simulink model "ClosedLoopTest"  (R2023a)
settings: Solver=VariableStepAuto  StartTime=0.0  StopTime=500  RelTol=1e-3
undefined symbols (not defined in the file): B, I, J, Ke, Kt, La, Ra, RW_omega_max, T_ext, T_max
libraries: simulink_extras x7, matrix_library x5, slpidlib x3, simulink x2, vrlib x2, aerolibutil x1
settings Model: Creator=Personal  LastModifiedBy=Personal
settings OptimizationCC: ReuseModelBlockBuffer=off
settings DebuggingCC: UnderSpecifiedDimensionMsg=warning

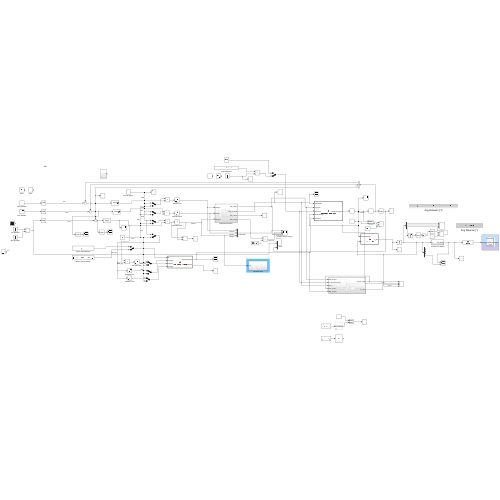
[thumbnail: Simulink's stored preview of the top-level diagram]
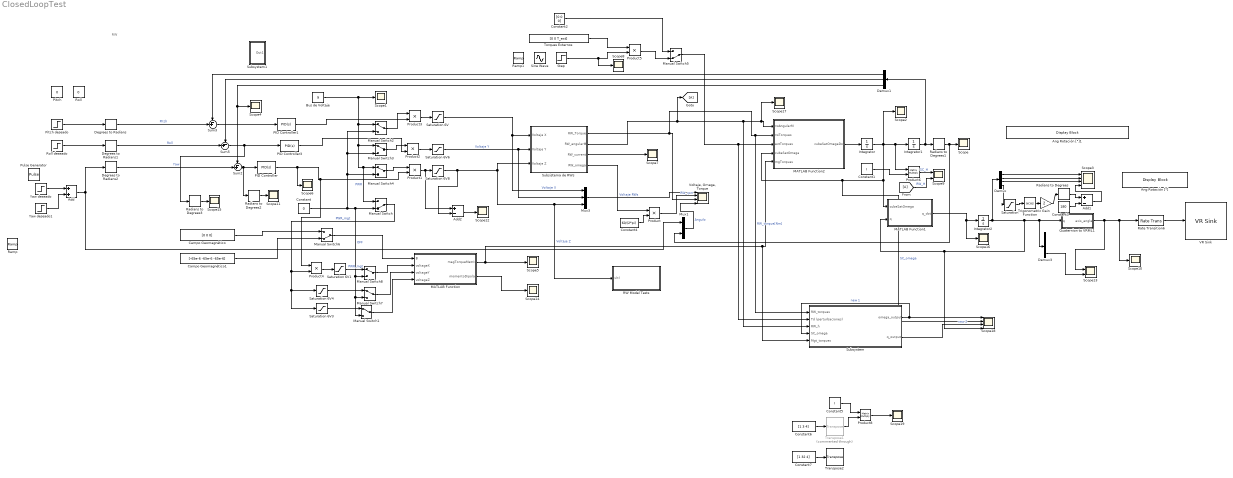
== system ClosedLoopTest ==
  note: RW
  Add : Sum
  Add1 : Sum  Inputs=+-
  Add2 : Sum  Inputs=+-
  Ang Rotación [°] : DisplayBlock  LabelPosition=Hide  Transparency=1
  Ang Rotación [°]1 : DisplayBlock  LabelPosition=Hide  Transparency=1
  Bus de Voltaje : Constant  Value=9
  Campo Geomagnético : Constant  Value=[0 0 0]
  Campo Geomagnético1 : Constant  Value=[-65e-6 -65e-6 -65e-6]
  Constant : Constant  Value=0
  Constant1 : Constant  Value=I
  Constant2 : Constant  Value=[0 0 0]
  Constant3 : Constant  Value=180
  Constant4 : Constant  Value=60/(2*pi)
  Constant5 : Constant  Value=I
  Constant6 : Constant  Value=[1 3 4]
  Constant7 : Constant  Value=[1 32 4]
  Degrees to Radians : simulink_extras/Transformations/Degrees to Radians
  Degrees to Radians1 : simulink_extras/Transformations/Degrees to Radians
  Degrees to Radians2 : simulink_extras/Transformations/Degrees to Radians
  Demux : Demux
  Demux1 : Demux  Outputs=3
  Demux3 : Demux
  From : From
  Gain : Gain  Gain=2
  Goto : Goto
  Integrator : Integrator  InitialCondition=[0 0 0]
  Integrator1 : Integrator  InitialCondition=[0 0 0]
  Integrator2 : Integrator  InitialCondition=[0 0 0 1]
  MATLAB Function : MATLAB Function  TreatAsAtomicUnit=on
  MATLAB Function1 : MATLAB Function  TreatAsAtomicUnit=on
  MATLAB Function2 : MATLAB Function  TreatAsAtomicUnit=on
  Manual Switch : ManualSwitch  CurrentSetting=0
  Manual Switch{1..4,7..8} (6 alike) : ManualSwitch
  Manual Switch5 : ManualSwitch  CurrentSetting=0
  Manual Switch6 : ManualSwitch  CurrentSetting=0
  Mux1 : Mux  Inputs=2
  Mux3 : Mux  Inputs=3
  PID Controller : slpidlib/PID Controller  Controller=PID  Form=Parallel  TimeDomain=Continuous-time  UseExternalTs=off  SampleTime=-1  IntegratorMethod=Forward Euler  FilterMethod=Forward Euler  ControllerParametersSource=internal  P=4500  I=800  UseKiTs=off  D=8000  N=100  UseFilter=on  TunerSelectOption=Transfer Function Based (PID Tuner App)  InitialConditionSource=internal  InitialConditionForIntegrator=0  InitialConditionForFilter=0  DifferentiatorICPrevScaledInput=0  ExternalReset=none  TrackingMode=off  Kt=1  LimitOutput=off  SatLimitsSource=internal  UpperSaturationLimit=1  LowerSaturationLimit=-1  LinearizeAsGain=on  AntiWindupMode=none  Kb=1  LimitIntegrator=off  UpperIntegratorSaturationLimit=inf  LowerIntegratorSaturationLimit=-inf  POutMin=[]  POutMax=[]  IOutMin=[]  IOutMax=[]  DOutMin=[]  DOutMax=[]  NOutMin=[]  NOutMax=[]  SumOutMin=[]  SumOutMax=[]  SaturationOutMin=[]  SaturationOutMax=[]  PParamMin=[]  PParamMax=[]  IParamMin=[]  IParamMax=[]  DParamMin=[]  DParamMax=[]  NParamMin=[]  NParamMax=[]  KbParamMin=[]  KbParamMax=[]  KtParamMin=[]  KtParamMax=[]  KbOutMin=[]  KbOutMax=[]  KtOutMin=[]  KtOutMax=[]  IntegratorOutMin=[]  IntegratorOutMax=[]  FilterOutMin=[]  FilterOutMax=[]  SumI1OutMin=[]  SumI1OutMax=[]  SumI2OutMin=[]  SumI2OutMax=[]  SumI3OutMin=[]  SumI3OutMax=[]  SumI4OutMin=[]  SumI4OutMax=[]  SumDOutMin=[]  SumDOutMax=[]  DifferentiatorOutMin=[]  DifferentiatorOutMax=[]  FilterDiffOutCoefMin=[]  FilterDiffOutCoefMax=[]  ReciprocalOutMin=[]  ReciprocalOutMax=[]  SumDenOutMin=[]  SumDenOutMax=[]  SumNumOutMin=[]  SumNumOutMax=[]  DivideOutMin=[]  DivideOutMax=[]  UdiffTsProdOutMin=[]  UdiffTsProdOutMax=[]  NTsProdOutMin=[]  NTsProdOutMax=[]  UintegralTsProdOutMin=[]  UintegralTsProdOutMax=[]  UngainTsProdOutMin=[]  UngainTsProdOutMax=[]  ClampingZeroOutDataTypeStr=Inherit: Inherit via back propagation  ClampingZeroOutMin=[]  ClampingZeroOutMax=[]  FilterDenConstantOutDataTypeStr=Inherit: Inherit via back propagation  FilterDenConstantOutMin=[]  FilterDenConstantOutMax=[]  PCopyOutDataTypeStr=Inherit: Inherit via back propagation  PCopyOutMin=[]  PCopyOutMax=[]  NCopyOutDataTypeStr=Inherit: Inherit via back propagation  NCopyOutMin=[]  NCopyOutMax=[]  IntegratorContinuousStateAttributes=''  IntegratorStateMustResolveToSignalObject=off  IntegratorRTWStateStorageClass=Auto  FilterContinuousStateAttributes=''  FilterStateMustResolveToSignalObject=off  FilterRTWStateStorageClass=Auto  ParallelPVariant=InternalParameters  IdealPVariant=Disabled  IVariant=InternalParameters  DVariant=InternalParameters  IntegratorVariant=Continuous  SatVariant=Disabled  AWVariant=Passthrough  PCopyVariant=Disabled  TRVariant=Disabled  FdbkBlocksVariant=Forward  IdealPFdbkVariant=Disabled  SatFdbkVariant=Disabled  DerivativeFilterVariant=ContFilter  NVariant=InternalParameters  NCopyVariant=Disabled  FilterICVariant=InternalICsFilter  IntegratorICVariant=InternalICs  ExternalResetVariant=Disabled  TRSumVariant=Passthrough  SumFdbkVariant=Disabled  SumVariant=Sum_PID  TsampFilterVariant=InternalTs  TsampNgainVariant=Passthrough  TsampIntegralVariant=Disabled_SignalSpec  ExternalSaturationOutDataTypeStr=Inherit: Same as second input
  PID Controller1 : slpidlib/PID Controller  Controller=PID  Form=Parallel  TimeDomain=Continuous-time  UseExternalTs=off  SampleTime=-1  IntegratorMethod=Forward Euler  FilterMethod=Forward Euler  ControllerParametersSource=internal  P=4500  I=800  UseKiTs=off  D=8000  N=100  UseFilter=on  TunerSelectOption=Transfer Function Based (PID Tuner App)  InitialConditionSource=internal  InitialConditionForIntegrator=0  InitialConditionForFilter=0  DifferentiatorICPrevScaledInput=0  ExternalReset=none  TrackingMode=off  Kt=1  LimitOutput=on  SatLimitsSource=internal  UpperSaturationLimit=1  LowerSaturationLimit=-1  LinearizeAsGain=on  AntiWindupMode=none  Kb=1  LimitIntegrator=off  UpperIntegratorSaturationLimit=inf  LowerIntegratorSaturationLimit=-inf  POutMin=[]  POutMax=[]  IOutMin=[]  IOutMax=[]  DOutMin=[]  DOutMax=[]  NOutMin=[]  NOutMax=[]  SumOutMin=[]  SumOutMax=[]  SaturationOutMin=[]  SaturationOutMax=[]  PParamMin=[]  PParamMax=[]  IParamMin=[]  IParamMax=[]  DParamMin=[]  DParamMax=[]  NParamMin=[]  NParamMax=[]  KbParamMin=[]  KbParamMax=[]  KtParamMin=[]  KtParamMax=[]  KbOutMin=[]  KbOutMax=[]  KtOutMin=[]  KtOutMax=[]  IntegratorOutMin=[]  IntegratorOutMax=[]  FilterOutMin=[]  FilterOutMax=[]  SumI1OutMin=[]  SumI1OutMax=[]  SumI2OutMin=[]  SumI2OutMax=[]  SumI3OutMin=[]  SumI3OutMax=[]  SumI4OutMin=[]  SumI4OutMax=[]  SumDOutMin=[]  SumDOutMax=[]  DifferentiatorOutMin=[]  DifferentiatorOutMax=[]  FilterDiffOutCoefMin=[]  FilterDiffOutCoefMax=[]  ReciprocalOutMin=[]  ReciprocalOutMax=[]  SumDenOutMin=[]  SumDenOutMax=[]  SumNumOutMin=[]  SumNumOutMax=[]  DivideOutMin=[]  DivideOutMax=[]  UdiffTsProdOutMin=[]  UdiffTsProdOutMax=[]  NTsProdOutMin=[]  NTsProdOutMax=[]  UintegralTsProdOutMin=[]  UintegralTsProdOutMax=[]  UngainTsProdOutMin=[]  UngainTsProdOutMax=[]  ClampingZeroOutDataTypeStr=Inherit: Inherit via back propagation  ClampingZeroOutMin=[]  ClampingZeroOutMax=[]  FilterDenConstantOutDataTypeStr=Inherit: Inherit via back propagation  FilterDenConstantOutMin=[]  FilterDenConstantOutMax=[]  PCopyOutDataTypeStr=Inherit: Inherit via back propagation  PCopyOutMin=[]  PCopyOutMax=[]  NCopyOutDataTypeStr=Inherit: Inherit via back propagation  NCopyOutMin=[]  NCopyOutMax=[]  IntegratorContinuousStateAttributes=''  IntegratorStateMustResolveToSignalObject=off  IntegratorRTWStateStorageClass=Auto  FilterContinuousStateAttributes=''  FilterStateMustResolveToSignalObject=off  FilterRTWStateStorageClass=Auto  ParallelPVariant=InternalParameters  IdealPVariant=Disabled  IVariant=InternalParameters  DVariant=InternalParameters  IntegratorVariant=Continuous  SatVariant=Enabled  AWVariant=Passthrough  PCopyVariant=Disabled  TRVariant=Disabled  FdbkBlocksVariant=Forward  IdealPFdbkVariant=Disabled  SatFdbkVariant=Disabled  DerivativeFilterVariant=ContFilter  NVariant=InternalParameters  NCopyVariant=Disabled  FilterICVariant=InternalICsFilter  IntegratorICVariant=InternalICs  ExternalResetVariant=Disabled  TRSumVariant=Passthrough  SumFdbkVariant=Disabled  SumVariant=Sum_PID  TsampFilterVariant=InternalTs  TsampNgainVariant=Passthrough  TsampIntegralVariant=Disabled_SignalSpec  ExternalSaturationOutDataTypeStr=Inherit: Same as second input
  PID Controller3 : slpidlib/PID Controller  Controller=PID  Form=Parallel  TimeDomain=Continuous-time  UseExternalTs=off  SampleTime=-1  IntegratorMethod=Forward Euler  FilterMethod=Forward Euler  ControllerParametersSource=internal  P=4500  I=800  UseKiTs=off  D=8000  N=100  UseFilter=on  TunerSelectOption=Transfer Function Based (PID Tuner App)  InitialConditionSource=internal  InitialConditionForIntegrator=0  InitialConditionForFilter=0  DifferentiatorICPrevScaledInput=0  ExternalReset=none  TrackingMode=off  Kt=1  LimitOutput=on  SatLimitsSource=internal  UpperSaturationLimit=1  LowerSaturationLimit=-1  LinearizeAsGain=on  AntiWindupMode=none  Kb=1  LimitIntegrator=off  UpperIntegratorSaturationLimit=inf  LowerIntegratorSaturationLimit=-inf  POutMin=[]  POutMax=[]  IOutMin=[]  IOutMax=[]  DOutMin=[]  DOutMax=[]  NOutMin=[]  NOutMax=[]  SumOutMin=[]  SumOutMax=[]  SaturationOutMin=[]  SaturationOutMax=[]  PParamMin=[]  PParamMax=[]  IParamMin=[]  IParamMax=[]  DParamMin=[]  DParamMax=[]  NParamMin=[]  NParamMax=[]  KbParamMin=[]  KbParamMax=[]  KtParamMin=[]  KtParamMax=[]  KbOutMin=[]  KbOutMax=[]  KtOutMin=[]  KtOutMax=[]  IntegratorOutMin=[]  IntegratorOutMax=[]  FilterOutMin=[]  FilterOutMax=[]  SumI1OutMin=[]  SumI1OutMax=[]  SumI2OutMin=[]  SumI2OutMax=[]  SumI3OutMin=[]  SumI3OutMax=[]  SumI4OutMin=[]  SumI4OutMax=[]  SumDOutMin=[]  SumDOutMax=[]  DifferentiatorOutMin=[]  DifferentiatorOutMax=[]  FilterDiffOutCoefMin=[]  FilterDiffOutCoefMax=[]  ReciprocalOutMin=[]  ReciprocalOutMax=[]  SumDenOutMin=[]  SumDenOutMax=[]  SumNumOutMin=[]  SumNumOutMax=[]  DivideOutMin=[]  DivideOutMax=[]  UdiffTsProdOutMin=[]  UdiffTsProdOutMax=[]  NTsProdOutMin=[]  NTsProdOutMax=[]  UintegralTsProdOutMin=[]  UintegralTsProdOutMax=[]  UngainTsProdOutMin=[]  UngainTsProdOutMax=[]  ClampingZeroOutDataTypeStr=Inherit: Inherit via back propagation  ClampingZeroOutMin=[]  ClampingZeroOutMax=[]  FilterDenConstantOutDataTypeStr=Inherit: Inherit via back propagation  FilterDenConstantOutMin=[]  FilterDenConstantOutMax=[]  PCopyOutDataTypeStr=Inherit: Inherit via back propagation  PCopyOutMin=[]  PCopyOutMax=[]  NCopyOutDataTypeStr=Inherit: Inherit via back propagation  NCopyOutMin=[]  NCopyOutMax=[]  IntegratorContinuousStateAttributes=''  IntegratorStateMustResolveToSignalObject=off  IntegratorRTWStateStorageClass=Auto  FilterContinuousStateAttributes=''  FilterStateMustResolveToSignalObject=off  FilterRTWStateStorageClass=Auto  ParallelPVariant=InternalParameters  IdealPVariant=Disabled  IVariant=InternalParameters  DVariant=InternalParameters  IntegratorVariant=Continuous  SatVariant=Enabled  AWVariant=Passthrough  PCopyVariant=Disabled  TRVariant=Disabled  FdbkBlocksVariant=Forward  IdealPFdbkVariant=Disabled  SatFdbkVariant=Disabled  DerivativeFilterVariant=ContFilter  NVariant=InternalParameters  NCopyVariant=Disabled  FilterICVariant=InternalICsFilter  IntegratorICVariant=InternalICs  ExternalResetVariant=Disabled  TRSumVariant=Passthrough  SumFdbkVariant=Disabled  SumVariant=Sum_PID  TsampFilterVariant=InternalTs  TsampNgainVariant=Passthrough  TsampIntegralVariant=Disabled_SignalSpec  ExternalSaturationOutDataTypeStr=Inherit: Same as second input
  Pitch : Constant  Value=0
  Pitch deseado : Step  Time=5  After=0  SampleTime=0
  Product{,1..5} (6 alike) : Product
  Product6 : Product  Multiplication=Matrix(*)
  Product8 : Product  Multiplication=Matrix(*)
  Pulse Generator : DiscretePulseGenerator  PulseType=Time based  Amplitude=45  Period=20  PulseWidth=50
  Quaternion to VRML1 : Subsystem
  RW Model Tests : Subsystem
  Radians to Degrees{,1..3} (4 alike) : simulink_extras/Transformations/Radians to Degrees
  Ramp : simulink/Sources/Ramp  slope=5  start=0  InitialOutput=0
  Ramp1 : simulink/Sources/Ramp  slope=2  start=3  InitialOutput=0
  Rate Transition6 : RateTransition
  Roll : Constant  Value=0
  Roll deseado : Step  Time=5  After=0  SampleTime=0
  Saturation : Saturate  UpperLimit=1  LowerLimit=-1
  Saturation 6V{,3,6,8} (4 alike) : Saturate  UpperLimit=6  LowerLimit=-6
  Saturation 6V1 : Saturate  UpperLimit=5  LowerLimit=-5
  Saturation 6V4 : Saturate  UpperLimit=2  LowerLimit=-6
  Scope{,1..2,4..8,10..12,14..17,19} (16 alike) : Scope
  Scope13 : Scope  NumInputPorts=2
  Scope18 : Scope  NumInputPorts=4
  Scope3 : Scope  NumInputPorts=4
  Scope9 : Scope  NumInputPorts=2
  Sine Wave : Sin  Amplitude=1.5  Frequency=0.01  SampleTime=0
  Step : Step  Time=0  After=100  SampleTime=0
  "Subsistema de RWs  " : Subsystem
  Subsystem : Subsystem
  Subsystem1 : Subsystem
  Sum2 : Sum  Inputs=-+|
  Sum3 : Sum  Inputs=-+|
  Sum5 : Sum  Inputs=-+|
  Torques Externos : Constant  Value=[0 0 T_ext]
  Transpose1 : matrix_library/Transpose  Commented=through
  Transpose2 : matrix_library/Transpose
  Trigonometric Function : Trigonometry  Operator=acos
  VR Sink : vrlib/VR Sink  InstantiateOnLoad=on  SampleTime=0.1  ViewEnable=on  RemoteChange=off  RemoteView=off  FieldsWritten=STLB_Transform.rotation.4.1.1.double  WorldFileName=EscenarioCubeSat.x3d  AutoView=off  VideoDimensions=[]  AllowVariableSize=off
  "Voltaje, Omega, Torque" : Scope  NumInputPorts=4
  Yaw deseado : Step  Time=5  After=45  SampleTime=0
  Yaw deseado1 : Step  Time=15  After=0  SampleTime=0
  wires:
  Saturation 6V/1 -> Mux3/1, "Subsistema de RWs  "/1(Voltaje X)  "Voltaje X"
  Saturation 6V6/1 -> "Subsistema de RWs  "/2(Voltaje Y), Mux3/2  "Voltaje Y"
  Saturation 6V8/1 -> Add2/2, "Subsistema de RWs  "/3(Voltaje Z), RW Model Tests/1(v(t)), Mux3/3  "Voltaje Z"
  MATLAB Function2/1(cubeSatOmegaDot) -> Integrator/1
  Integrator/1 -> Product6/1, Integrator1/1, Scope18/2, MATLAB Function2/4(cubeSatOmega), MATLAB Function1/1(cubeSatOmega), Scope2/1  "SC_omega"
  Integrator1/1 -> Demux1/1, Radians to Degrees1/1
  MATLAB Function/1(magTorqueMatrix) -> Subsystem/5(Mgt_torques), MATLAB Function2/5(mgTorques), Scope5/1
  Constant/1 -> Manual Switch2/2, Manual Switch3/2, Manual Switch4/2, Manual Switch1/2, Manual Switch7/2, Manual Switch8/2, Manual Switch/2  "OFF"
  Saturation 6V3/1 -> Manual Switch1/1
  Manual Switch1/1 -> MATLAB Function/4(voltageZ)
  Manual Switch5/1 -> Subsystem/2(Td (perturbaciones)), MATLAB Function2/3(extTorques)
  Constant2/1 -> Manual Switch5/1
  Manual Switch6/1 -> MATLAB Function/1(B)
  Campo Geomagnético/1 -> Manual Switch6/1
  Campo Geomagnético1/1 -> Manual Switch6/2
  Saturation 6V4/1 -> Manual Switch7/1
  Manual Switch/1 -> Saturation 6V4/1, Saturation 6V3/1, Product4/2  "PWR_mgt"
  Manual Switch8/1 -> MATLAB Function/2(voltageX)
  Manual Switch7/1 -> MATLAB Function/3(voltageY)
  MATLAB Function1/1(q_dot) -> Scope16/1, Integrator2/1
  Integrator2/1 -> Quaternion to VRML1/1(q), Demux3/1, Scope18/4, MATLAB Function1/2(q), Demux/1
  Demux/1 -> Scope3/1
  Demux/2 -> Scope3/2
  Demux/3 -> Scope3/3
  Radians to Degrees/1 -> Add1/1
  Radians to Degrees1/1 -> Mux1/2, Scope/1
  Demux/4 -> Saturation/1
  Trigonometric Function/1 -> Gain/1
  Gain/1 -> Radians to Degrees/1
  Quaternion to VRML1/1(axis_angle) -> Scope13/1, Scope10/1, Rate Transition6/1
  Constant3/1 -> Add1/2
  Add1/1 -> Scope3/4
  Bus de Voltaje/1 -> Manual Switch2/1, Manual Switch3/1, Manual Switch/1, Manual Switch4/1, Scope1/1  "PWR"
  MATLAB Function/2(momentoDipolar) -> Scope14/1
  Constant4/1 -> Product/2
  Product/1 -> "Voltaje, Omega, Torque"/2  "RW_rpm"
  Demux3/4 -> Scope13/2
  Rate Transition6/1 -> VR Sink/1
  Saturation/1 -> Trigonometric Function/1
  Add/1 -> Degrees to Radians2/1, Mux1/1
  Degrees to Radians/1 -> Sum3/2  "Pitch"
  Degrees to Radians2/1 -> Sum2/2  "Yaw"
  Degrees to Radians1/1 -> Sum5/2  "Roll"
  Demux1/1 -> Sum3/1
  Demux1/2 -> Sum5/1
  Demux1/3 -> Scope4/1, Sum2/1
  Manual Switch4/1 -> Product1/1
  Product1/1 -> Add2/1, Saturation 6V8/1
  Sum3/1 -> PID Controller1/1
  Product3/1 -> Saturation 6V/1
  Product2/1 -> Saturation 6V6/1
  Manual Switch3/1 -> Product2/1
  Manual Switch2/1 -> Product3/1
  PID Controller1/1 -> Product3/2
  PID Controller3/1 -> Product2/2
  Radians to Degrees2/1 -> Scope11/1
  Product4/1 -> Saturation 6V1/1
  Saturation 6V1/1 -> Manual Switch8/1  "PWR_mgt"
  PID Controller/1 -> Scope6/1, Product1/2, Product4/1
  Sum2/1 -> PID Controller/1, Radians to Degrees2/1
  Torques Externos/1 -> Product5/1
  Step/1 -> Scope8/1, Product5/2
  Product5/1 -> Manual Switch5/2
  Sum5/1 -> Radians to Degrees3/1, PID Controller3/1
  Radians to Degrees3/1 -> Scope15/1
  Roll deseado/1 -> Degrees to Radians1/1
  Pitch deseado/1 -> Degrees to Radians/1
  Mux3/1 -> "Voltaje, Omega, Torque"/1  "Voltaje RWs"
  "Subsistema de RWs  "/2(RW_angularM) -> Goto/1, Subsystem/3(RW_h), Scope17/1, MATLAB Function2/1(rwAngularM)
  "Subsistema de RWs  "/4(RW_omega) -> Product/1
  "Subsistema de RWs  "/1(RW_Torque) -> Subsystem/1(RW_torques), MATLAB Function2/2(rwTorques), "Voltaje, Omega, Torque"/3  "RW_torque[Nm]"
  "Subsistema de RWs  "/3(RW_current) -> Scope7/1
  Mux1/1 -> "Voltaje, Omega, Torque"/4  "Angulo"
  Constant1/1 -> Product6/2
  Product6/1 -> Scope9/1  "SC_H"
  From/1 -> Scope9/2  "RW_H"
  Yaw deseado/1 -> Add/1
  Yaw deseado1/1 -> Add/2
  Add2/1 -> Scope12/1
  Subsystem/1(omega_output) -> Scope18/1, Subsystem/4(SC_omega)  "new 1"
  Subsystem/2(q_output) -> Scope18/3  "new 2"
  Constant5/1 -> Product8/1
  Transpose1/1 -> Product8/2
  Constant6/1 -> Transpose1/1
  Product8/1 -> Scope19/1
  Constant7/1 -> Transpose2/1

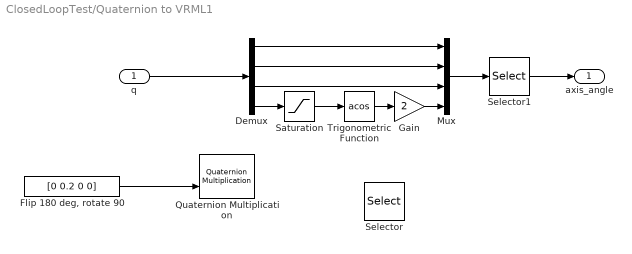
== system ClosedLoopTest/Quaternion to VRML1 ==
  q : Inport
  Demux : Demux
  "Flip 180 deg, rotate 90" : Constant  Value=[0 0.2 0 0]
  Gain : Gain  Gain=2
  Mux : Mux
  Quaternion Multiplication : aerolibutil/Quaternion Multiplication
  Saturation : Saturate  UpperLimit=1  LowerLimit=-1  ZeroCross=off
  Selector : Selector  InputPortWidth=3  IndexOptions=Index vector (dialog)  Indices=[1 3]  OutputSizes=1
  Selector1 : Selector  InputPortWidth=4  IndexOptions=Index vector (dialog)  Indices=[2 3 1 4]  OutputSizes=1
  Trigonometric Function : Trigonometry  Operator=acos
  axis_angle : Outport  VectorParamsAs1DForOutWhenUnconnected=off
  wires:
  Demux/2 -> Mux/2
  "Flip 180 deg, rotate 90"/1 -> Quaternion Multiplication/2
  q/1 -> Demux/1
  Demux/1 -> Mux/1
  Mux/1 -> Selector1/1
  Selector1/1 -> axis_angle/1
  Trigonometric Function/1 -> Gain/1
  Gain/1 -> Mux/4
  Demux/3 -> Mux/3
  Saturation/1 -> Trigonometric Function/1
  Demux/4 -> Saturation/1

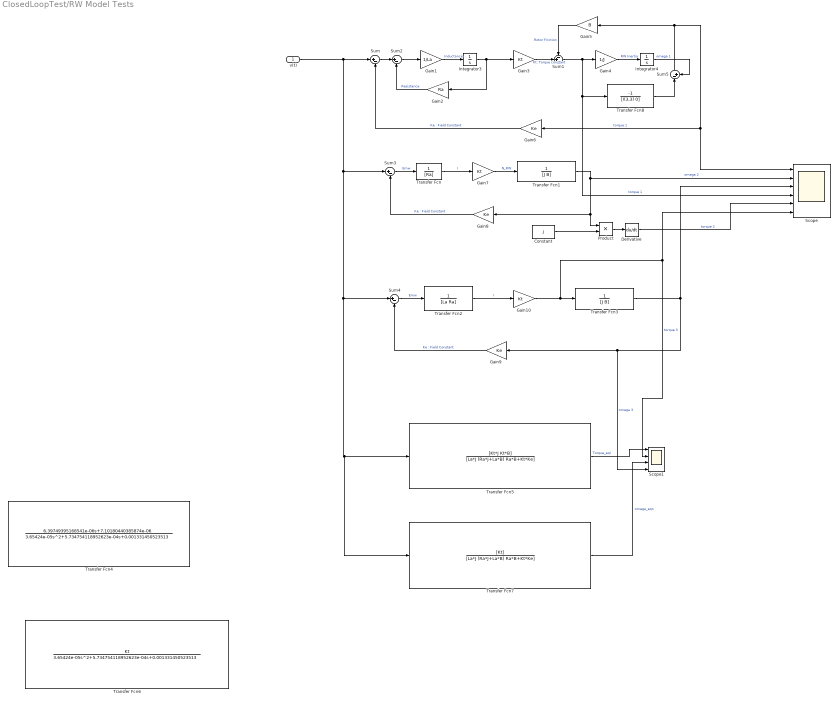
== system ClosedLoopTest/RW Model Tests ==
  v(t) : Inport
  Constant : Constant  Value=J
  Derivative : Derivative
  Gain1 : Gain  Gain=1/La
  Gain10 : Gain  Gain=Kt
  Gain2 : Gain  Gain=Ra
  Gain3 : Gain  Gain=Kt
  Gain4 : Gain  Gain=1/J
  Gain5 : Gain  Gain=B
  Gain6 : Gain  Gain=Ke
  Gain7 : Gain  Gain=Kt
  Gain8 : Gain  Gain=Ke
  Gain9 : Gain  Gain=Ke
  Integrator3 : Integrator
  Integrator4 : Integrator
  Product : Product
  Scope : Scope  NumInputPorts=6
  Scope1 : Scope  NumInputPorts=4
  Sum{,2..4} (4 alike) : Sum  Inputs=|+-
  Sum1 : Sum  Inputs=-+|
  Sum5 : Sum  Inputs=|-+
  Transfer Fcn : TransferFcn  Denominator=[Ra]
  Transfer Fcn1 : TransferFcn  Denominator=[J B]
  Transfer Fcn2 : TransferFcn  Denominator=[La Ra]
  Transfer Fcn3 : TransferFcn  Denominator=[J B]
  Transfer Fcn4 : TransferFcn  Numerator=[6.39749395168541e-06 7.10180440385874e-06]  Denominator=[3.65424e-05 5.734754118952623e-04 0.001331450523513]
  Transfer Fcn5 : TransferFcn  Numerator=[Kt*J Kt*B]  Denominator=[La*J (Ra*J+La*B) Ra*B+Kt*Ke]
  Transfer Fcn6 : TransferFcn  Numerator=Kt  Denominator=[3.65424e-05 5.734754118952623e-04 0.001331450523513]
  Transfer Fcn7 : TransferFcn  Numerator=[Kt]  Denominator=[La*J (Ra*J+La*B) Ra*B+Kt*Ke]
  Transfer Fcn8 : TransferFcn  Numerator=[-1]  Denominator=[I(3,3) 0]
  wires:
  Sum1/1 -> Gain4/1, Transfer Fcn8/1, Scope/4  "torque 1"
  Derivative/1 -> Scope/5  "torque 2"
  Transfer Fcn3/1 -> Scope/3, Gain9/1, Scope1/4  "omega 3"
  Gain10/1 -> Transfer Fcn3/1, Scope/6, Scope1/2  "torque 3"
  Transfer Fcn2/1 -> Gain10/1  "I"
  Gain9/1 -> Sum4/2  "Ke : Field Constant"
  Sum4/1 -> Transfer Fcn2/1  "Emw"
  Gain2/1 -> Sum2/2  "Resistance"
  Integrator3/1 -> Gain2/1, Gain3/1
  Gain6/1 -> Sum/2  "Ke : Field Constant"
  Gain5/1 -> Sum1/1  "Rotor Friction"
  Sum2/1 -> Gain1/1
  Integrator4/1 -> Sum5/2  "omega 1"
  Gain4/1 -> Integrator4/1  "RW Inertia"
  Gain1/1 -> Integrator3/1  "Inductance"
  Gain3/1 -> Sum1/2  "Kt: Torque constant"
  Sum/1 -> Sum2/1
  v(t)/1 -> Transfer Fcn7/1, Transfer Fcn5/1, Sum4/1, Sum3/1, Sum/1
  Sum3/1 -> Transfer Fcn/1  "Emw"
  Gain7/1 -> Transfer Fcn1/1  "N_RW"
  Transfer Fcn/1 -> Gain7/1  "I"
  Transfer Fcn1/1 -> Product/1, Gain8/1, Scope/2  "omega 2"
  Gain8/1 -> Sum3/2  "Ke : Field Constant"
  Product/1 -> Derivative/1
  Constant/1 -> Product/2
  Transfer Fcn5/1 -> Scope1/1  "Torque_eqI"
  Transfer Fcn7/1 -> Scope1/3  "omega_eqn"
  Transfer Fcn8/1 -> Sum5/1
  Sum5/1 -> Gain5/1, Scope/1, Gain6/1  "torque 1"

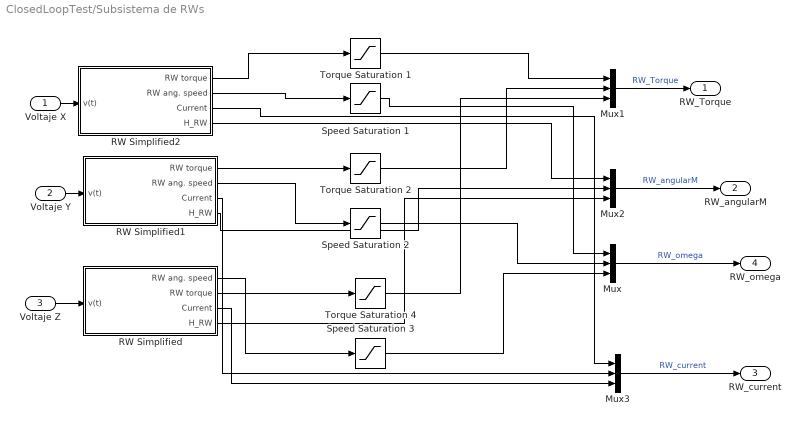
== system ClosedLoopTest/Subsistema de RWs   ==
  Voltaje X : Inport
  Voltaje Y : Inport  Port=2
  Voltaje Z : Inport  Port=3
  Mux{,1..3} (4 alike) : Mux  Inputs=3
  RW Simplified : Subsystem
  RW Simplified1 : Subsystem
  RW Simplified2 : Subsystem
  Speed Saturation 1 : Saturate  UpperLimit=RW_omega_max  LowerLimit=-RW_omega_max
  Speed Saturation 2 : Saturate  UpperLimit=RW_omega_max  LowerLimit=-RW_omega_max
  Speed Saturation 3 : Saturate  UpperLimit=RW_omega_max  LowerLimit=-RW_omega_max
  Torque Saturation 1 : Saturate  UpperLimit=T_max  LowerLimit=-T_max
  Torque Saturation 2 : Saturate  UpperLimit=T_max  LowerLimit=-T_max
  Torque Saturation 4 : Saturate  UpperLimit=T_max  LowerLimit=-T_max
  RW_Torque : Outport
  RW_angularM : Outport  Port=2
  RW_current : Outport  Port=3
  RW_omega : Outport  Port=4
  wires:
  RW Simplified/2(RW torque) -> Torque Saturation 4/1
  RW Simplified2/1(RW torque) -> Torque Saturation 1/1
  Torque Saturation 4/1 -> Mux1/3
  Voltaje Z/1 -> RW Simplified/1(v(t))
  Speed Saturation 2/1 -> Mux/2
  RW Simplified1/1(RW torque) -> Torque Saturation 2/1
  RW Simplified/4(H_RW) -> Mux2/3
  Mux1/1 -> RW_Torque/1  "RW_Torque"
  Voltaje X/1 -> RW Simplified2/1(v(t))
  Speed Saturation 1/1 -> Mux/1
  RW Simplified1/4(H_RW) -> Mux2/2
  Speed Saturation 3/1 -> Mux/3
  Voltaje Y/1 -> RW Simplified1/1(v(t))
  RW Simplified1/2(RW ang. speed) -> Speed Saturation 2/1
  RW Simplified2/4(H_RW) -> Mux2/1
  RW Simplified2/2(RW ang. speed) -> Speed Saturation 1/1
  RW Simplified/1(RW ang. speed) -> Speed Saturation 3/1
  Torque Saturation 2/1 -> Mux1/2
  Mux2/1 -> RW_angularM/1  "RW_angularM"
  Torque Saturation 1/1 -> Mux1/1
  Mux/1 -> RW_omega/1  "RW_omega"
  RW Simplified/3(Current) -> Mux3/3
  RW Simplified1/3(Current) -> Mux3/2
  Mux3/1 -> RW_current/1  "RW_current"
  RW Simplified2/3(Current) -> Mux3/1

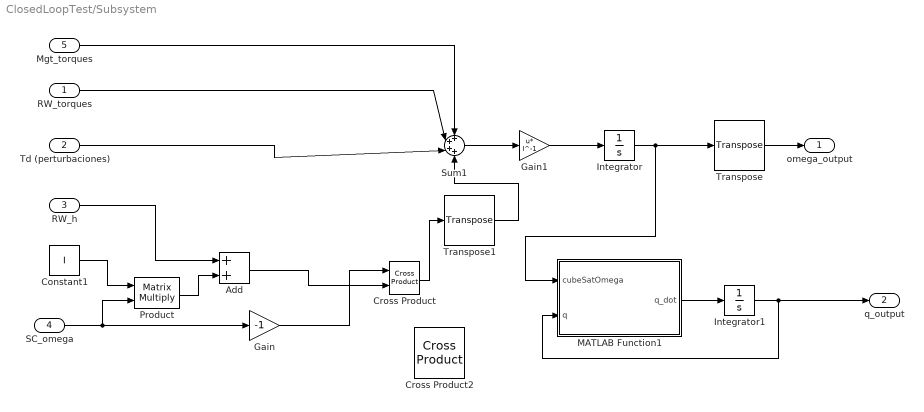
== system ClosedLoopTest/Subsystem ==
  RW_torques : Inport
  Td (perturbaciones) : Inport  Port=2
  RW_h : Inport  Port=3
  SC_omega : Inport  Port=4
  Mgt_torques : Inport  Port=5
  Add : Sum
  Constant1 : Constant  Value=I
  Cross Product : vrlib/Utilities/Cross Product
  Cross Product2 : matrix_library/Cross Product
  Gain : Gain  Gain=-1
  Gain1 : Gain  Gain=I^-1  Multiplication=Matrix(u*K)
  Integrator : Integrator  InitialCondition=[0 0 0]
  Integrator1 : Integrator  InitialCondition=[0 0 0 1]
  MATLAB Function1 : MATLAB Function  TreatAsAtomicUnit=on
  Product : Product  Multiplication=Matrix(*)
  Sum1 : Sum  Inputs=++++
  Transpose : matrix_library/Transpose
  Transpose1 : matrix_library/Transpose
  omega_output : Outport
  q_output : Outport  Port=2
  wires:
  RW_torques/1 -> Sum1/2
  Td (perturbaciones)/1 -> Sum1/3
  Integrator1/1 -> MATLAB Function1/2(q), q_output/1
  Constant1/1 -> Product/1
  Product/1 -> Add/2
  RW_h/1 -> Add/1
  Gain/1 -> Cross Product/1
  Add/1 -> Cross Product/2
  Cross Product/1 -> Transpose1/1
  Sum1/1 -> Gain1/1
  Gain1/1 -> Integrator/1
  Integrator/1 -> MATLAB Function1/1(cubeSatOmega), Transpose/1
  MATLAB Function1/1(q_dot) -> Integrator1/1
  Mgt_torques/1 -> Sum1/1
  SC_omega/1 -> Product/2, Gain/1
  Transpose/1 -> omega_output/1
  Transpose1/1 -> Sum1/4

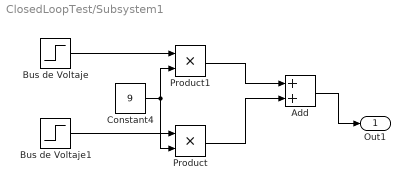
== system ClosedLoopTest/Subsystem1 ==
  Add : Sum
  Bus de Voltaje : Step  Time=3  SampleTime=0
  Bus de Voltaje1 : Step  Time=5  After=-1  SampleTime=0
  Constant4 : Constant  Value=9
  Product : Product
  Product1 : Product
  Out1 : Outport
  wires:
  Bus de Voltaje1/1 -> Product/1
  Add/1 -> Out1/1
  Product1/1 -> Add/1
  Product/1 -> Add/2
  Constant4/1 -> Product1/2, Product/2
  Bus de Voltaje/1 -> Product1/1

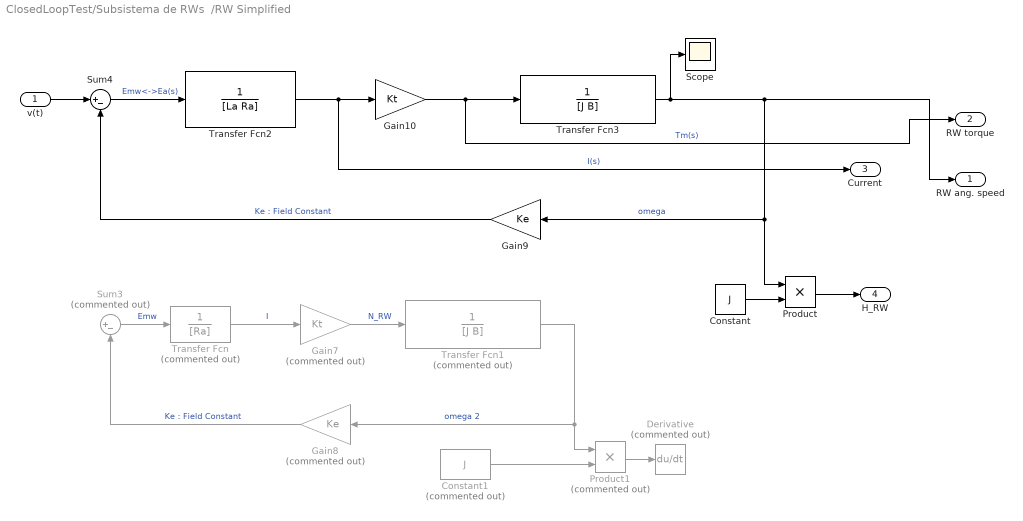
== system ClosedLoopTest/Subsistema de RWs  /RW Simplified ==
  v(t) : Inport
  Constant : Constant  Value=J
  Constant1 : Constant  Commented=on  Value=J
  Derivative : Derivative  Commented=on
  Gain10 : Gain  Gain=Kt
  Gain7 : Gain  Commented=on  Gain=Kt
  Gain8 : Gain  Commented=on  Gain=Ke
  Gain9 : Gain  Gain=Ke
  Product : Product
  Product1 : Product  Commented=on
  Scope : Scope
  Sum3 : Sum  Commented=on  Inputs=|+-
  Sum4 : Sum  Inputs=|+-
  Transfer Fcn : TransferFcn  Commented=on  Denominator=[Ra]
  Transfer Fcn1 : TransferFcn  Commented=on  Denominator=[J B]
  Transfer Fcn2 : TransferFcn  Denominator=[La Ra]
  Transfer Fcn3 : TransferFcn  Denominator=[J B]
  RW ang. speed : Outport  VectorParamsAs1DForOutWhenUnconnected=off
  RW torque : Outport  Port=2  VectorParamsAs1DForOutWhenUnconnected=off
  Current : Outport  Port=3  VectorParamsAs1DForOutWhenUnconnected=off
  H_RW : Outport  Port=4  VectorParamsAs1DForOutWhenUnconnected=off
  wires:
  Gain10/1 -> RW torque/1, Transfer Fcn3/1  "Tm(s)"
  Transfer Fcn2/1 -> Current/1, Gain10/1  "I(s)"
  Sum4/1 -> Transfer Fcn2/1  "Emw<->Ea(s)"
  Gain9/1 -> Sum4/2  "Ke : Field Constant"
  Transfer Fcn3/1 -> Scope/1, Gain9/1, Product/1, RW ang. speed/1  "omega"
  Constant/1 -> Product/2
  Product/1 -> H_RW/1
  v(t)/1 -> Sum4/1
  Product1/1 -> Derivative/1
  Constant1/1 -> Product1/2
  Transfer Fcn1/1 -> Product1/1, Gain8/1  "omega 2"
  Gain7/1 -> Transfer Fcn1/1  "N_RW"
  Sum3/1 -> Transfer Fcn/1  "Emw"
  Transfer Fcn/1 -> Gain7/1  "I"
  Gain8/1 -> Sum3/2  "Ke : Field Constant"

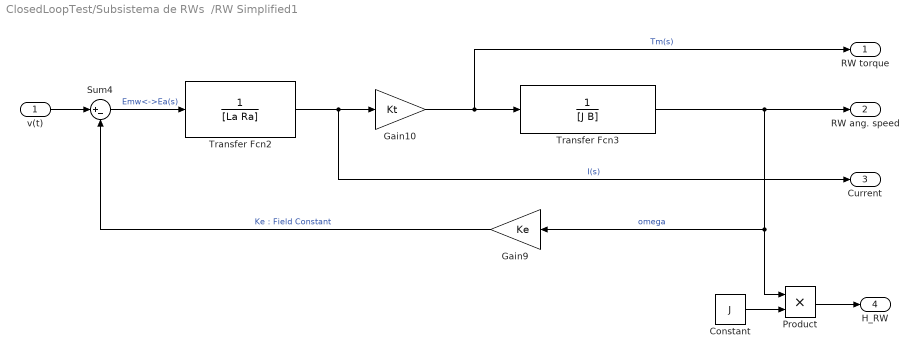
== system ClosedLoopTest/Subsistema de RWs  /RW Simplified1 ==
  v(t) : Inport
  Constant : Constant  Value=J
  Gain10 : Gain  Gain=Kt
  Gain9 : Gain  Gain=Ke
  Product : Product
  Sum4 : Sum  Inputs=|+-
  Transfer Fcn2 : TransferFcn  Denominator=[La Ra]
  Transfer Fcn3 : TransferFcn  Denominator=[J B]
  RW torque : Outport  VectorParamsAs1DForOutWhenUnconnected=off
  RW ang. speed : Outport  Port=2  VectorParamsAs1DForOutWhenUnconnected=off
  Current : Outport  Port=3  VectorParamsAs1DForOutWhenUnconnected=off
  H_RW : Outport  Port=4  VectorParamsAs1DForOutWhenUnconnected=off
  wires:
  Product/1 -> H_RW/1
  Constant/1 -> Product/2
  Transfer Fcn3/1 -> Product/1, Gain9/1, RW ang. speed/1  "omega"
  Gain9/1 -> Sum4/2  "Ke : Field Constant"
  Sum4/1 -> Transfer Fcn2/1  "Emw<->Ea(s)"
  Transfer Fcn2/1 -> Gain10/1, Current/1  "I(s)"
  Gain10/1 -> Transfer Fcn3/1, RW torque/1  "Tm(s)"
  v(t)/1 -> Sum4/1

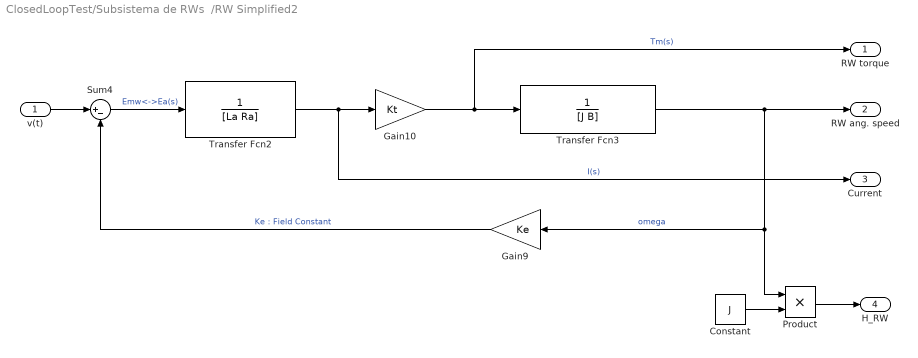
== system ClosedLoopTest/Subsistema de RWs  /RW Simplified2 ==
  v(t) : Inport
  Constant : Constant  Value=J
  Gain10 : Gain  Gain=Kt
  Gain9 : Gain  Gain=Ke
  Product : Product
  Sum4 : Sum  Inputs=|+-
  Transfer Fcn2 : TransferFcn  Denominator=[La Ra]
  Transfer Fcn3 : TransferFcn  Denominator=[J B]
  RW torque : Outport  VectorParamsAs1DForOutWhenUnconnected=off
  RW ang. speed : Outport  Port=2  VectorParamsAs1DForOutWhenUnconnected=off
  Current : Outport  Port=3  VectorParamsAs1DForOutWhenUnconnected=off
  H_RW : Outport  Port=4  VectorParamsAs1DForOutWhenUnconnected=off
  wires:
  v(t)/1 -> Sum4/1
  Gain10/1 -> RW torque/1, Transfer Fcn3/1  "Tm(s)"
  Transfer Fcn2/1 -> Current/1, Gain10/1  "I(s)"
  Sum4/1 -> Transfer Fcn2/1  "Emw<->Ea(s)"
  Gain9/1 -> Sum4/2  "Ke : Field Constant"
  Transfer Fcn3/1 -> RW ang. speed/1, Gain9/1, Product/1  "omega"
  Constant/1 -> Product/2
  Product/1 -> H_RW/1

== matlab function ClosedLoopTest/MATLAB Function1 ==
  data: cubeSatOmega input; q_dot output; q input
function q_dot = omega2qdot(cubeSatOmega,q)

wx = cubeSatOmega(1);
wy = cubeSatOmega(2);
wz = cubeSatOmega(3);

OmegaMatrix = [0 wz -wy wx ;
               -wz 0 wx wy; 
               wy -wx 0 wz;
               -wx -wy -wz 0];
            
q_dot=0.5*OmegaMatrix*q;

end

== matlab function ClosedLoopTest/MATLAB Function ==
  data: B input; magTorqueMatrix output; voltageX input; voltageY input; voltageZ input; momentoDipolar output
function [magTorqueMatrix,momentoDipolar] = magTorqueFunction(B,voltageX,voltageY,voltageZ)

%d = 1.45e-2; % Diametro mgt [m]
d = 2e-2; % Diametro mgt [m]
A =d^2*pi/4;

mu_0 = 1.25663706212e-6; % Permeabilidad del vacío [Vs/Am]
mu_r = 200000; % Permeabilidad del relativa del Hierro [-] Ref-> http://hyperphysics.phy-astr.gsu.edu/hbase/Tables/magprop.html#c2
L = 0.585; % H % Impedancia [H] 
%L = 11.2534e-3; % Impedancia [H] 
l = 7.92e-2; % Longitud mgt [m] 

%n=sqrt(L*l/(mu_0*mu_r*A)); % # Vueltas 
n = 5412;

%R = 50.7 ;% Resistencia mgt [Ohm];
R = 30 ;% Resistencia mgt [Ohm];
ix = voltageX/R;
iy = voltageY/R;
iz = voltageZ/R;

% M = [n*ix*A n*iy*A n*iz*A]';
% 
% magTorqueMatrix = -skew(B)*M;

magTorqueMatrix_X = cross(n*ix*A*[1 0 0],B);
magTorqueMatrix_Y = cross(n*iy*A*[0 1 0],B);
magTorqueMatrix_Z = cross(n*iz*A*[0 0 1],B);
 momentoDipolar = [n*ix*A n*iy*A n*iz*A];

magTorqueMatrix = magTorqueMatrix_X+magTorqueMatrix_Y+magTorqueMatrix_Z;

== matlab function ClosedLoopTest/MATLAB Function2 ==
  data: rwAngularM input; rwTorques input; cubeSatOmegaDot output size=[1 3]; extTorques input; cubeSatOmega input size=3; mgTorques input
function cubeSatOmegaDot  = cubeSatDynamicModel(rwAngularM,rwTorques,extTorques,cubeSatOmega,mgTorques)

% Inercia EyasSat [kg m2]
I =1e-7*[336109.715 0 0 ;
        0 308250.765 0; 
        0 0 271714.972];

% % Inercia EyasSat [kg m2]
% I =1e-7*[335592.028 0 0 ;
%         0 335592.028 0; 
%         0 0 335592.028];

%Momentos de inercia EyasSat
Ixx = I(1,1);
Iyy = I(2,2);
Izz = I(3,3);

%Velocidades angulares EyasSat
wx = cubeSatOmega(1);
wy = cubeSatOmega(2);
wz = cubeSatOmega(3);

%Torques externos
Tx = extTorques(1);
Ty = extTorques(2);
Tz = extTorques(3);

%Torques de control RW
Tc_x = rwTorques(1);
Tc_y = rwTorques(2);
Tc_z = rwTorques(3);

%Torques de control RW
Tmg_x = mgTorques(1);
Tmg_y = mgTorques(2);
Tmg_z = mgTorques(3);

hx = rwAngularM(1);
hy = rwAngularM(2);
hz = rwAngularM(3);



omegaDotX = (Tx+Tc_x+Tmg_x+wy*wz*(Iyy-Izz)-hz*wy+hy*wz)/Ixx;
omegaDotY = (Ty+Tc_y+Tmg_y+wx*wz*(Izz-Ixx)-hx*wz+hz*wx)/Iyy;
omegaDotZ = (Tz+Tc_z+Tmg_z+wx*wy*(Ixx-Iyy)-hy*wx+hx*wy)/Izz;

cubeSatOmegaDot = [omegaDotX omegaDotY omegaDotZ];

== matlab function ClosedLoopTest/Subsystem/MATLAB Function1 ==
  data: cubeSatOmega input; q_dot output; q input
function q_dot = omega2qdot(cubeSatOmega,q)

wx = cubeSatOmega(1);
wy = cubeSatOmega(2);
wz = cubeSatOmega(3);

OmegaMatrix = [0 wz -wy wx ;
               -wz 0 wx wy; 
               wy -wx 0 wz;
               -wx -wy -wz 0];
            
q_dot=0.5*OmegaMatrix*q;

end
